simulink model "demonstration"  (R2022a)
settings: Solver=ode1be  StartTime=0.0  StopTime=1.5  FixedStep=1e-4  RelTol=1e-3
model workspace (MAT data in the model file):
  Consum = [12000 18000 24000 30000 36000 42000 48000]
libraries: kif2 x14, spsRMSLib x14, SignalEditorBlockLib x2, spsGroundLib x1, eePowerMeasurement x1, spsThreePhaseProgrammableVoltageSourceLib x1, spsThreePhaseSeriesRLCBranchLib x1, spsThreePhaseSeriesRLCLoadLib x1, spspowerguiLib x1
settings Model: Creator=Felhasználó  LastModifiedBy=Felhasználó

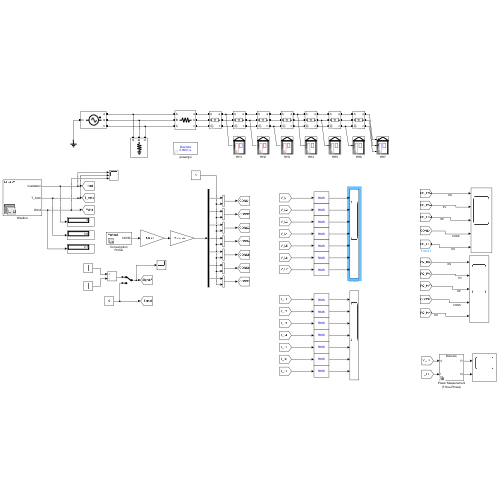
[thumbnail: Simulink's stored preview of the top-level diagram]
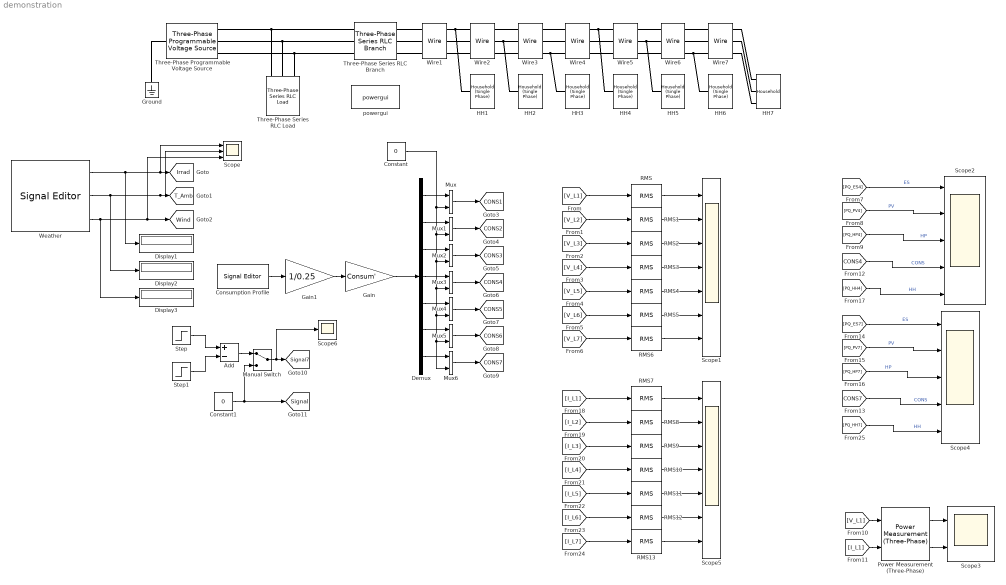
== system demonstration ==
  Add : Sum  Inputs=+-
  Constant : Constant  Value=0
  Constant1 : Constant  Value=0
  Consumption Profile : SignalEditorBlockLib/Signal Editor  FileName=CONS24.mat  ActiveScenario=Munka1  ActiveSignal=CONS  IsBus=off  OutputBusObjectStr=Bus: BusObject  SampleTime=0  ZeroCross=off  OutputAfterFinalValue=Setting to zero  Unit=inherit  PreserveSignalName=on
  Demux : Demux  Outputs=7
  Display1 : Display
  Display2 : Display
  Display3 : Display
  Gain : Gain  Gain=Consum'
  Gain1 : Gain  Gain=1/0.25
  Ground : spsGroundLib/Ground  LConnTagsString=a
  HH1 : kif2/Household (Single Phase)  Ctag=CONS1  Atag=Signal  Itag=Irrad  Ttag=T_Amb  Wtag=Wind  HHtag=PQ_HH1  HHtagv=global  PVtag=PQ_PV1  PVtagv=global  EStag=PQ_ES1  EStagv=global  HPtag=PQ_HP1  HPtagv=global
      link override ES: Cap=109600  SoCin=0.2  Pin=49400  Pout=-49400
      link override HP: P_HP=2400  Tset=21  C=2655  H=140
      link override PV: P_STCm=9200
      settings: SourceProductName=KIF2 Library
  HH2 : kif2/Household (Single Phase)  Ctag=CONS2  Atag=Signal  Itag=Irrad  Ttag=T_Amb  Wtag=Wind  HHtag=PQ_HH2  HHtagv=global  PVtag=PQ_PV2  PVtagv=global  EStag=PQ_ES2  EStagv=global  HPtag=PQ_HP2  HPtagv=global
      link override ES: Cap=164400  SoCin=0.3  Pin=73500  Pout=-73500
      link override HP: P_HP=3000  Tset=21  C=4950  H=141
      link override PV: P_STCm=13800
      settings: SourceProductName=KIF2 Library
  HH3 : kif2/Household (Single Phase)  Ctag=CONS3  Atag=Signal  Itag=Irrad  Ttag=T_Amb  Wtag=Wind  HHtag=PQ_HH3  HHtagv=global  PVtag=PQ_PV3  PVtagv=global  EStag=PQ_ES3  EStagv=global  HPtag=PQ_HP3  HPtagv=global
      link override ES: Cap=219200  SoCin=0.4  Pin=97600  Pout=-97600
      link override HP: P_HP=2500  Tset=21  C=2520  H=146
      link override PV: P_STCm=18500
      settings: SourceProductName=KIF2 Library
  HH4 : kif2/Household (Single Phase)  Ctag=CONS4  Atag=Signal  Itag=Irrad  Ttag=T_Amb  Wtag=Wind  HHtag=PQ_HH4  HHtagv=global  PVtag=PQ_PV4  PVtagv=global  EStag=PQ_ES4  EStagv=global  HPtag=PQ_HP4  HPtagv=global
      link override ES: Cap=274000  Pin=121600  Pout=-121600
      link override HP: P_HP=3300  Tset=21  C=4635  H=176
      link override PV: P_STCm=23100
      settings: SourceProductName=KIF2 Library
  HH5 : kif2/Household (Single Phase)  Ctag=CONS5  Atag=Signal  Itag=Irrad  Ttag=T_Amb  Wtag=Wind  HHtag=PQ_HH5  HHtagv=global  PVtag=PQ_PV5  PVtagv=global  EStag=PQ_ES5  EStagv=global  HPtag=PQ_HP5  HPtagv=global
      link override ES: Cap=328800  SoCin=0.6  Pin=145700  Pout=-145700
      link override HP: Tset=21
      link override PV: P_STCm=27700
      settings: SourceProductName=KIF2 Library
  HH6 : kif2/Household (Single Phase)  Ctag=CONS6  Atag=Signal  Itag=Irrad  Ttag=T_Amb  Wtag=Wind  HHtag=PQ_HH6  HHtagv=global  PVtag=PQ_PV6  PVtagv=global  EStag=PQ_ES6  EStagv=global  HPtag=PQ_HP6  HPtagv=global
      link override ES: Cap=383600  SoCin=0.7  Pin=169800  Pout=-169800
      link override HP: P_HP=4200  Tset=21  C=4590  H=241
      settings: SourceProductName=KIF2 Library
  HH7 : kif2/Household  Ctag=CONS7  Atag=Signal7  Itag=Irrad  Ttag=T_Amb  Wtag=Wind  HHtag=PQ_HH7  HHtagv=global  PVtag=PQ_PV7  PVtagv=global  EStag=PQ_ES7  EStagv=global  HPtag=PQ_HP7  HPtagv=global
      link override ES: Cap=438400  SoCin=0.8  Pin=193800  Pout=-193800
      link override HP: P_HP=4800  Tset=21  C=5220  H=284
      link override PV: P_STCm=36900
      settings: SourceProductName=KIF2 Library
  Manual Switch : ManualSwitch
  Mux{,1..6} (7 alike) : RealImagToComplex
  Power Measurement (Three-Phase) : eePowerMeasurement/Power Measurement (Three-Phase)  LabelModeActiveChoice=Discrete  F=50  K=[1]  Seq=Positive  Ts=1e-4
      settings: SourceProductBaseCode=PS
  RMS{,1..13} (14 alike) : spsRMSLib/RMS  TrueRMS=on  Freq=50  RMSInit=230  Ts=0
  Scope : Scope  NumInputPorts=3
  Scope1 : Scope  NumInputPorts=7
  Scope2 : Scope  NumInputPorts=5
  Scope3 : Scope  NumInputPorts=2
  Scope4 : Scope  NumInputPorts=5
  Scope5 : Scope  NumInputPorts=7
  Scope6 : Scope
  Step : Step  Time=0.5  After=-1  SampleTime=0
  Step1 : Step  After=-1  SampleTime=0
  Three-Phase Programmable Voltage Source : spsThreePhaseProgrammableVoltageSourceLib/Three-Phase Programmable Voltage Source  PositiveSequence="[400  0 50]"  VariationEntity=None  VariationType=Modulation  VariationTypeAlt=Step  VariationStep=0.5  VariationRate=10  VariationMagnitude=0.3  VariationFrequency=2  VariationTiming=[100 1000]  VariationPhaseA=off  Amplitudes=[1 0.8 1.2 1.0]  TimeValues=[0 0.1 0.15 0.2]  HarmonicGeneration=off  HarmonicA=[3 0.2 -25 0]  HarmonicB=[2 0.15 35 2]  Timing="[0.05  3]"  BusType=swing  Pref=0  Qref=0  Qmin=-inf  Qmax=inf
  Three-Phase Series RLC Branch : spsThreePhaseSeriesRLCBranchLib/Three-Phase Series RLC Branch  LConnTagsString=A|B|C  RConnTagsString=A|B|C  BranchType=R  Resistance=0.001  Inductance=1e-3  Capacitance=1e-6  Measurements=None
  Three-Phase Series RLC Load : spsThreePhaseSeriesRLCLoadLib/Three-Phase Series RLC Load  LConnTagsString=A|B|C  Configuration=Y (grounded)  NominalVoltage=400  Vabc=[1e3 1e3 1e3]  Vabcp=[1e3 1e3 1e3]  NominalFrequency=50  UnbalancedPower=off  ActivePower=10e3  InductivePower=0  CapacitivePower=0  Pabc=[10e3 9e3 11e3]  QLabc=[100 90 110]  QCabc=[100 90 110]  Pabcp=[10e3 9e3 11e3]  QLabcp=[100 90 110]  QCabcp=[100 90 110]  Measurements=None  LoadType=constant Z
  Weather : SignalEditorBlockLib/Signal Editor  FileName=irrad24.mat  ActiveScenario=Munka2  ActiveSignal=Irradiation  IsBus=off  OutputBusObjectStr=Bus: BusObject  SampleTime=0  ZeroCross=off  OutputAfterFinalValue=Setting to zero  Unit=inherit  PreserveSignalName=on
  Wire1 : kif2/Wire  Length=0.12  Frequency=50  Resistances=[296.8421e-003 446.8421e-003]  Inductances=[953.5880e-006 5.4671e-003]  Capacitances=[12.4583e-009 3.9055e-009]  Vtag=V_L1  Vtagv=global  Itag=I_L1  Itagv=global
      settings: SourceProductName=KIF2 Library
  Wire2 : kif2/Wire  Length=0.12  Frequency=50  Resistances=[296.8421e-003 446.8421e-003]  Inductances=[953.5880e-006 5.4671e-003]  Capacitances=[12.4583e-009 3.9055e-009]  Vtag=V_L2  Vtagv=global  Itag=I_L2  Itagv=global
      settings: SourceProductName=KIF2 Library
  Wire3 : kif2/Wire  Length=0.12  Frequency=50  Resistances=[296.8421e-003 446.8421e-003]  Inductances=[953.5880e-006 5.4671e-003]  Capacitances=[12.4583e-009 3.9055e-009]  Vtag=V_L3  Vtagv=global  Itag=I_L3  Itagv=global
      settings: SourceProductName=KIF2 Library
  Wire4 : kif2/Wire  Length=0.12  Frequency=50  Resistances=[296.8421e-003 446.8421e-003]  Inductances=[953.5880e-006 5.4671e-003]  Capacitances=[12.4583e-009 3.9055e-009]  Vtag=V_L4  Vtagv=global  Itag=I_L4  Itagv=global
      settings: SourceProductName=KIF2 Library
  Wire5 : kif2/Wire  Length=0.12  Frequency=50  Resistances=[296.8421e-003 446.8421e-003]  Inductances=[953.5880e-006 5.4671e-003]  Capacitances=[12.4583e-009 3.9055e-009]  Vtag=V_L5  Vtagv=global  Itag=I_L5  Itagv=global
      settings: SourceProductName=KIF2 Library
  Wire6 : kif2/Wire  Length=0.12  Frequency=50  Resistances=[296.8421e-003 446.8421e-003]  Inductances=[953.5880e-006 5.4671e-003]  Capacitances=[12.4583e-009 3.9055e-009]  Vtag=V_L6  Vtagv=global  Itag=I_L6  Itagv=global
      settings: SourceProductName=KIF2 Library
  Wire7 : kif2/Wire  Length=0.12  Frequency=50  Resistances=[296.8421e-003 446.8421e-003]  Inductances=[953.5880e-006 5.4671e-003]  Capacitances=[12.4583e-009 3.9055e-009]  Vtag=V_L7  Vtagv=global  Itag=I_L7  Itagv=global
      settings: SourceProductName=KIF2 Library
  powergui : spspowerguiLib/powergui  Priority=1  SimulationMode=Discrete  SampleTime=1e-4  frequency=60  Iterations=50  frequencyindice=50  Pbase=100e6  ErrMax=1e-4  UnitsV=kV  UnitsW=MW  buscounter=0  FunctionMessages=off  echomessages=off  EnableUseOfTLC=off  CurrentSourceSwitches=off  DisableSnubberDevices=off  DisableRonSwitches=off  DisableVfSwitches=off  DisplayEquations=off  AutomaticDiscreteSolvers=off  SolverType=Backward Euler  Interpol=off  ExternalGateDelay=off  methode=off  Ts=100  x0status=blocks  SPID=on  SwTol=0  HookPort=off  NonlinearTolerance=1e-4  nMaxIteration=100  ContinueOnMaxIteration=off  RestoreLinks=warning  ResistiveCurrentMeasurement=off  Frange=[0:2:500]  Ylog=off  Xlog=on  ShowGrid=off  save=off  variable=ZData  structure=0  ZoomFFT=off  StartTime=0.0  cycles=1  DisplayStyle=1  fundamental=60  FreqAxis=off  MaxFrequency=1000  frequencyindicesteady=1  RmsSteady=1  display=off
  tag scope: CONS1=global, CONS2=global, CONS3=global, CONS4=global, CONS5=global, CONS6=global, CONS7=global, Irrad=global, Signal7=global, Signal=global, T_Amb=global, Wind=global
  wires:
  [PQ_HP7] -> Scope4/3  "HP"
  Demux/1 -> Mux/1
  RMS3/1 -> Scope1/4
  [CONS4] -> Scope2/4  "CONS"
  Power Measurement (Three-Phase)/2 -> Scope3/2
  Gain/1 -> Demux/1
  Demux/4 -> Mux3/1
  Mux4/1 -> [CONS5]
  [PQ_ES7] -> Scope4/1  "ES"
  [I_L1] -> Power Measurement (Three-Phase)/2
  Constant/1 -> Mux6/2, Mux5/2, Mux4/2, Mux3/2, Mux2/2, Mux1/2, Mux/2
  [PQ_PV7] -> Scope4/2  "PV"
  Gain1/1 -> Gain/1
  Constant1/1 -> Manual Switch/2, [Signal]
  [CONS7] -> Scope4/4  "CONS"
  Demux/3 -> Mux2/1
  RMS5/1 -> Scope1/6
  RMS1/1 -> Scope1/2
  RMS6/1 -> Scope1/7
  [V_L5] -> RMS4/1
  Consumption Profile/1 -> Gain1/1
  Mux6/1 -> [CONS7]
  Mux/1 -> [CONS1]
  [V_L2] -> RMS1/1
  Mux1/1 -> [CONS2]
  Demux/6 -> Mux5/1
  Weather/2 -> Display2/1, Scope/2, [T_Amb]
  [V_L1] -> RMS/1
  [V_L6] -> RMS5/1
  Demux/5 -> Mux4/1
  Mux2/1 -> [CONS3]
  [V_L4] -> RMS3/1
  Demux/7 -> Mux6/1
  [PQ_HP4] -> Scope2/3  "HP"
  Power Measurement (Three-Phase)/1 -> Scope3/1
  Demux/2 -> Mux1/1
  Weather/3 -> Display3/1, Scope/3, [Wind]
  [V_L7] -> RMS6/1
  Weather/1 -> Scope/1, [Irrad], Display1/1
  [V_L1] -> Power Measurement (Three-Phase)/1
  [V_L3] -> RMS2/1
  RMS2/1 -> Scope1/3
  RMS/1 -> Scope1/1
  [PQ_ES4] -> Scope2/1  "ES"
  RMS4/1 -> Scope1/5
  Mux5/1 -> [CONS6]
  Mux3/1 -> [CONS4]
  [PQ_PV4] -> Scope2/2  "PV"
  [PQ_HH4] -> Scope2/5  "HH"
  RMS11/1 -> Scope5/5
  RMS7/1 -> Scope5/1
  RMS9/1 -> Scope5/3
  [I_L3] -> RMS9/1
  [I_L7] -> RMS13/1
  [I_L4] -> RMS10/1
  [I_L6] -> RMS12/1
  [I_L1] -> RMS7/1
  [I_L2] -> RMS8/1
  [I_L5] -> RMS11/1
  RMS13/1 -> Scope5/7
  RMS8/1 -> Scope5/2
  RMS12/1 -> Scope5/6
  RMS10/1 -> Scope5/4
  Add/1 -> Manual Switch/1
  Manual Switch/1 -> Scope6/1, [Signal7]
  [PQ_HH7] -> Scope4/5  "HH"
  Step/1 -> Add/1
  Step1/1 -> Add/2
  connections:
  HH1/LConn1 -- Wire1/RConn1 -- Wire2/LConn1
  Wire1/RConn2 -- Wire2/LConn2
  Wire1/RConn3 -- Wire2/LConn3
  HH2/LConn1 -- Wire2/RConn2 -- Wire3/LConn2
  Wire2/RConn1 -- Wire3/LConn1
  Wire2/RConn3 -- Wire3/LConn3
  HH3/LConn1 -- Wire3/RConn3 -- Wire4/LConn3
  Wire3/RConn1 -- Wire4/LConn1
  Wire3/RConn2 -- Wire4/LConn2
  HH4/LConn1 -- Wire4/RConn1 -- Wire5/LConn1
  Wire4/RConn2 -- Wire5/LConn2
  Wire4/RConn3 -- Wire5/LConn3
  HH5/LConn1 -- Wire5/RConn2 -- Wire6/LConn2
  Wire5/RConn1 -- Wire6/LConn1
  Wire5/RConn3 -- Wire6/LConn3
  HH6/LConn1 -- Wire6/RConn3 -- Wire7/LConn3
  Wire6/RConn1 -- Wire7/LConn1
  Wire6/RConn2 -- Wire7/LConn2
  Wire7/RConn1 -- HH7/LConn1
  Wire7/RConn2 -- HH7/LConn2
  Wire7/RConn3 -- HH7/LConn3
  Three-Phase Series RLC Branch/LConn2 -- Three-Phase Programmable Voltage Source/RConn2 -- Three-Phase Series RLC Load/LConn2
  Three-Phase Series RLC Branch/LConn3 -- Three-Phase Series RLC Load/LConn3 -- Three-Phase Programmable Voltage Source/RConn3
  Three-Phase Series RLC Branch/LConn1 -- Three-Phase Programmable Voltage Source/RConn1 -- Three-Phase Series RLC Load/LConn1
  Wire1/LConn3 -- Three-Phase Series RLC Branch/RConn3
  Wire1/LConn2 -- Three-Phase Series RLC Branch/RConn2
  Three-Phase Programmable Voltage Source/LConn1 -- Ground/LConn1
  Wire1/LConn1 -- Three-Phase Series RLC Branch/RConn1
